simulink model "solar_panel_model"  (R2024b)
settings: Solver=VariableStepAuto  StartTime=0.0  StopTime=10.0  RelTol=1e-3
libraries: simulink x1
settings Model: Creator=paulin.kantue  LastModifiedBy=lerat
settings RTWCC: GPUComputeCapability=3.5

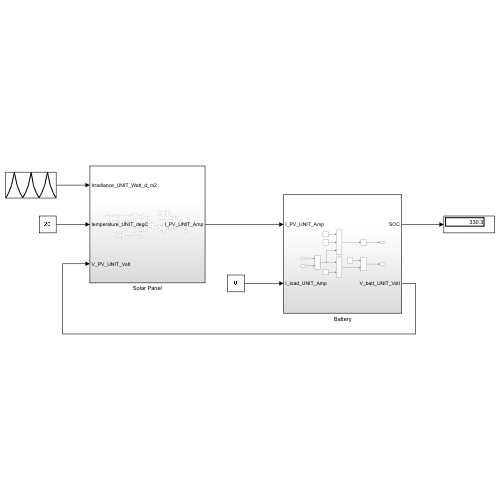
[thumbnail: Simulink's stored preview of the top-level diagram]
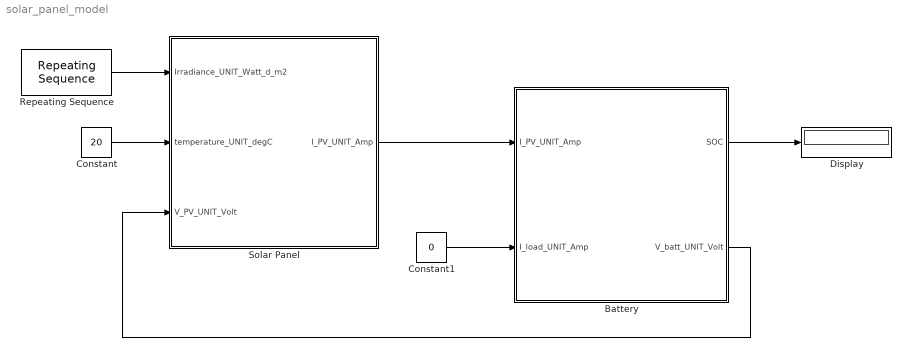
== system solar_panel_model ==
  Battery : Subsystem
  Constant : Constant  Value=20
  Constant1 : Constant  Value=0
  Display : Display
  Repeating Sequence : simulink/Sources/Repeating Sequence  rep_seq_t=[0 2 4 6 8 10 12]  rep_seq_y=[0 200 500 1000 500 200 0]
  Solar Panel : Subsystem
  wires:
  Solar Panel/1(I_PV_UNIT_Amp) -> Battery/1(I_PV_UNIT_Amp)
  Battery/1(SOC) -> Display/1
  Battery/2(V_batt_UNIT_Volt) -> Solar Panel/3(V_PV_UNIT_Volt)
  Repeating Sequence/1 -> Solar Panel/1(Irradiance_UNIT_Watt_d_m2)
  Constant/1 -> Solar Panel/2(temperature_UNIT_degC)
  Constant1/1 -> Battery/2(I_load_UNIT_Amp)

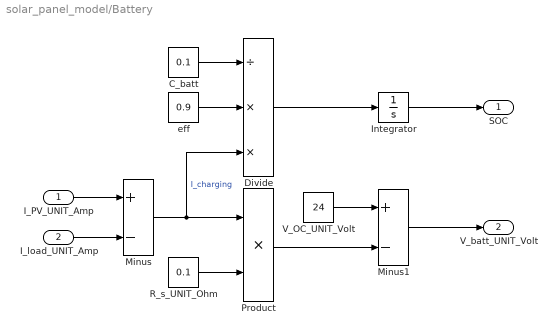
== system solar_panel_model/Battery ==
  I_PV_UNIT_Amp : Inport
  I_load_UNIT_Amp : Inport  Port=2
  C_batt : Constant  Value=0.1
  Divide : Product  Inputs=/**
  Integrator : Integrator
  Minus : Sum  Inputs=+-
  Minus1 : Sum  Inputs=+-
  Product : Product
  R_s_UNIT_Ohm : Constant  Value=0.1
  V_OC_UNIT_Volt : Constant  Value=24
  eff : Constant  Value=0.9
  SOC : Outport
  V_batt_UNIT_Volt : Outport  Port=2
  wires:
  Minus/1 -> Divide/3, Product/1  "I_charging"
  R_s_UNIT_Ohm/1 -> Product/2
  I_PV_UNIT_Amp/1 -> Minus/1
  I_load_UNIT_Amp/1 -> Minus/2
  Product/1 -> Minus1/2
  V_OC_UNIT_Volt/1 -> Minus1/1
  Minus1/1 -> V_batt_UNIT_Volt/1
  Integrator/1 -> SOC/1
  C_batt/1 -> Divide/1
  eff/1 -> Divide/2
  Divide/1 -> Integrator/1

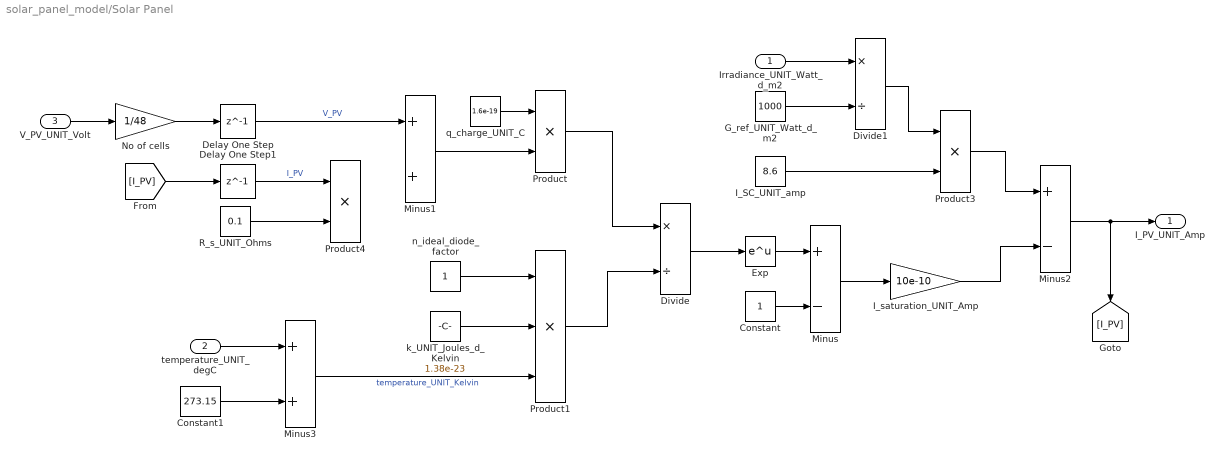
== system solar_panel_model/Solar Panel ==
  Irradiance_UNIT_Watt_d_m2 : Inport
  temperature_UNIT_degC : Inport  Port=2
  V_PV_UNIT_Volt : Inport  Port=3
  Constant : Constant
  Constant1 : Constant  Value=273.15
  Delay One Step : Delay  DelayLength=1
  Delay One Step1 : Delay  DelayLength=1
  Divide : Product  Inputs=*/
  Divide1 : Product  Inputs=*/
  Exp : Math
  G_ref_UNIT_Watt_d_m2 : Constant  Value=1000
  I_SC_UNIT_amp : Constant  Value=8.6
  I_saturation_UNIT_Amp : Gain  Gain=10e-10
  Minus : Sum  Inputs=+-
  Minus1 : Sum
  Minus2 : Sum  Inputs=+-
  Minus3 : Sum
  No of cells : Gain  Gain=1/48
  Product : Product
  Product1 : Product  Inputs=3
  Product3 : Product
  Product4 : Product
  R_s_UNIT_Ohms : Constant  Value=0.1
  k_UNIT_Joules_d_Kelvin : Constant  Value=1.38e-23
  n_ideal_diode_factor : Constant
  q_charge_UNIT_C : Constant  Value=1.6e-19
  I_PV_UNIT_Amp : Outport
  wires:
  q_charge_UNIT_C/1 -> Product/1
  Delay One Step/1 -> Minus1/1  "V_PV"
  k_UNIT_Joules_d_Kelvin/1 -> Product1/2
  n_ideal_diode_factor/1 -> Product1/1
  Minus3/1 -> Product1/3  "temperature_UNIT_Kelvin"
  Product1/1 -> Divide/2
  Divide/1 -> Exp/1
  Irradiance_UNIT_Watt_d_m2/1 -> Divide1/1
  G_ref_UNIT_Watt_d_m2/1 -> Divide1/2
  Delay One Step1/1 -> Product4/1  "I_PV"
  R_s_UNIT_Ohms/1 -> Product4/2
  Minus1/1 -> Product/2
  Product/1 -> Divide/1
  Exp/1 -> Minus/1
  Constant/1 -> Minus/2
  Minus/1 -> I_saturation_UNIT_Amp/1
  I_SC_UNIT_amp/1 -> Product3/2
  Divide1/1 -> Product3/1
  Product3/1 -> Minus2/1
  I_saturation_UNIT_Amp/1 -> Minus2/2
  Minus2/1 -> I_PV_UNIT_Amp/1, [I_PV]
  [I_PV] -> Delay One Step1/1
  temperature_UNIT_degC/1 -> Minus3/1
  Constant1/1 -> Minus3/2
  No of cells/1 -> Delay One Step/1
  V_PV_UNIT_Volt/1 -> No of cells/1
